simulink model "MSDR_DH_DeplV1sim"  (R2019a)
settings: Solver=ode45  StartTime=0.0  StopTime=simtime  FixedStep=0.1  MaxStep=ts_max  RelTol=rel_tolerance
values from neighbouring files (symbols this model uses):
  a_f = 1E-5*depl_fuel_temp_coef(depl_index)    [MSDR_DH_DeplV1para.m]
  a_g = 1E-5*depl_grap_temp_coef(depl_index)    [MSDR_DH_DeplV1para.m]
  A_s = 1.2245    [MSDR_DH_DeplV1para.m]
  beta = depl_beta(depl_index,:)    [MSDR_DH_DeplV1para.m]
  beta_t = sum(beta)    [MSDR_DH_DeplV1para.m]
  Cp_f = depl_Cp_Fuel_coef*1.355616e-3    [MSDR_DH_DeplV1para.m]
  Cp_p = Cp_s_shx    [MSDR_DH_DeplV1para.m]
  Cp_s = Cp_s*1e-6    (= 3.588208e-09)    [MSDR_DH_DeplV1para.m]
  Cp_sc = 4761.392e-6    (= 0.004761392)    [MSDR_DH_DeplV1para.m]
  Cp_w = 456.056e-6    (= 0.000456056)    [MSDR_DH_DeplV1para.m]
  D_it = 0.0141478    [MSDR_DH_DeplV1para.m]
  D_ot = 0.015875    [MSDR_DH_DeplV1para.m]
  DHRS_TIME_K = 10    [MSDR_DH_DeplV1para.m]
  dHs_dPs = -0.042433622114357    (= -0.0424336221144)    [MSDR_DH_DeplV1para.m]
  Epsilon = 1E-3    (= 0.001)    [MSDR_DH_DeplV1para.m]
  Fiss_factor = 2.464783802008740e-03    (= 0.00246478380201)    [MSDR_DH_DeplV1para.m]
  gamma0 = 9.635981959409105e-01    (= 0.963598195941)    [MSDR_DH_DeplV1para.m]
  gamma1 = 3.560674858154914e-02    (= 0.0356067485815)    [MSDR_DH_DeplV1para.m]
  gamma2 = 7.950554775404400e-04    (= 0.00079505547754)    [MSDR_DH_DeplV1para.m]
  gamma_I = 5.1135e-2    (= 0.051135)    [MSDR_DH_DeplV1para.m]
  gamma_Pm = 1.08E-2    (= 0.0108)    [MSDR_DH_DeplV1para.m]
  gamma_Xe = 1.1628e-2    (= 0.011628)    [MSDR_DH_DeplV1para.m]
  h_pw = h_s_shx    [MSDR_DH_DeplV1para.m]
  h_wb = 13349.334646671E-6    (= 0.0133493346467)    [MSDR_DH_DeplV1para.m]
  h_ws = 5732.378387768E-6    (= 0.00573237838777)    [MSDR_DH_DeplV1para.m]
  h_wsc = 8385.005556375E-6    (= 0.00838500555638)    [MSDR_DH_DeplV1para.m]
  hA_fg = [h_fg*A_fg/2, h_fg*A_fg/2]    [MSDR_DH_DeplV1para.m]
  hA_p_phx1 = h_p_phx*A_p_phx    [MSDR_DH_DeplV1para.m]
  hA_p_phx2 = h_p_phx*A_p_phx    [MSDR_DH_DeplV1para.m]
  hA_p_phx3 = h_p_phx*A_p_phx    [MSDR_DH_DeplV1para.m]
  hA_p_phx4 = h_p_phx*A_p_phx    [MSDR_DH_DeplV1para.m]
  hA_p_phx5 = h_p_phx*A_p_phx    [MSDR_DH_DeplV1para.m]
  hA_p_phx6 = h_p_phx*A_p_phx    [MSDR_DH_DeplV1para.m]
  hA_p_shx1 = h_p_shx*A_p_shx    [MSDR_DH_DeplV1para.m]
  hA_p_shx2 = h_p_shx*A_p_shx    [MSDR_DH_DeplV1para.m]
  hA_p_shx3 = h_p_shx*A_p_shx    [MSDR_DH_DeplV1para.m]
  hA_p_shx4 = h_p_shx*A_p_shx    [MSDR_DH_DeplV1para.m]
  hA_p_shx5 = h_p_shx*A_p_shx    [MSDR_DH_DeplV1para.m]
  hA_p_shx6 = h_p_shx*A_p_shx    [MSDR_DH_DeplV1para.m]
  hA_s_phx1 = h_s_phx*A_s_phx    [MSDR_DH_DeplV1para.m]
  hA_s_phx2 = h_s_phx*A_s_phx    [MSDR_DH_DeplV1para.m]
  hA_s_phx3 = h_s_phx*A_s_phx    [MSDR_DH_DeplV1para.m]
  hA_s_phx4 = h_s_phx*A_s_phx    [MSDR_DH_DeplV1para.m]
  hA_s_phx5 = h_s_phx*A_s_phx    [MSDR_DH_DeplV1para.m]
  hA_s_phx6 = h_s_phx*A_s_phx    [MSDR_DH_DeplV1para.m]
  hA_s_shx1 = h_s_shx*A_s_shx    [MSDR_DH_DeplV1para.m]
  hA_s_shx2 = h_s_shx*A_s_shx    [MSDR_DH_DeplV1para.m]
  hA_s_shx3 = h_s_shx*A_s_shx    [MSDR_DH_DeplV1para.m]
  hA_s_shx4 = h_s_shx*A_s_shx    [MSDR_DH_DeplV1para.m]
  hA_s_shx5 = h_s_shx*A_s_shx    [MSDR_DH_DeplV1para.m]
  hA_s_shx6 = h_s_shx*A_s_shx    [MSDR_DH_DeplV1para.m]
  I_0 = gamma_I*Sig_f_msdr*phi_0/lam_I    [MSDR_DH_DeplV1para.m]
  Ifa = [0.25, 0.25]    [MSDR_DH_DeplV1para.m]
  Ifb = [0.25, 0.25]    [MSDR_DH_DeplV1para.m]
  Ig = [0.5, 0.5]    [MSDR_DH_DeplV1para.m]
  K_1 = 11.632248097704855    (= 11.6322480977)    [MSDR_DH_DeplV1para.m]
  K_4 = b(1)    [MSDR_DH_DeplV1para.m]
  K_5 = a(1)    [MSDR_DH_DeplV1para.m]
  K_b = 12.834854076292217    (= 12.8348540763)    [MSDR_DH_DeplV1para.m]
  K_pump = 1/5    (= 0.2)    [MSDR_DH_DeplV1para.m]
  K_sc = -17.615718797133468    (= -17.6157187971)    [MSDR_DH_DeplV1para.m]
  ka = [0.235, 0.235]    [MSDR_DH_DeplV1para.m]
  kb = [0.235, 0.235]    [MSDR_DH_DeplV1para.m]
  kga = [0.015, 0.015]    [MSDR_DH_DeplV1para.m]
  kgb = [0.015, 0.015]    [MSDR_DH_DeplV1para.m]
  L = 8.5344    [MSDR_DH_DeplV1para.m]
  L_b = 2.3645    [MSDR_DH_DeplV1para.m]
  L_s = 4.723    [MSDR_DH_DeplV1para.m]
  Lam = depl_Lam(depl_index)    [MSDR_DH_DeplV1para.m]
  lam = [1.240E-02, 3.05E-02, 1.11E-01, 3.01E-01, 1.140E+00, 3.014E+00]    [MSDR_DH_DeplV1para.m]
  lam_bubl = 2.0e-2    (= 0.02)    [MSDR_DH_DeplV1para.m]
  lam_I = 2.875e-5    (= 2.875e-05)    [MSDR_DH_DeplV1para.m]
  lam_Pm = log(2)/(2.21*24*3600)    [MSDR_DH_DeplV1para.m]
  lam_Xe = 2.0916e-5    (= 2.0916e-05)    [MSDR_DH_DeplV1para.m]
  lambda0 = 0.0945298    [MSDR_DH_DeplV1para.m]
  lambda1 = 0.00441957    [MSDR_DH_DeplV1para.m]
  lambda2 = 8.60979e-05    [MSDR_DH_DeplV1para.m]
  m_3m = W_3*2    (= 8618.207327)    [MSDR_DH_DeplV1para.m]
  m_f_t = total_mp_phx + core_fm + mp_phxm*3 + m_fm    [MSDR_DH_DeplV1para.m]
  m_fm = W_f*1    (= 4989.48)    [MSDR_DH_DeplV1para.m]
  M_stm = 0.018    [MSDR_DH_DeplV1para.m]
  mcp_fa = mfa*Cp_f    [MSDR_DH_DeplV1para.m]
  mcp_fb = mfb*Cp_f    [MSDR_DH_DeplV1para.m]
  mcp_g = mg*Cp_g    [MSDR_DH_DeplV1para.m]
  mcp_p_phx1 = Cp_p_phx*mp_phx1    [MSDR_DH_DeplV1para.m]
  mcp_p_phx2 = Cp_p_phx*mp_phx2    [MSDR_DH_DeplV1para.m]
  mcp_p_phx3 = Cp_p_phx*mp_phx3    [MSDR_DH_DeplV1para.m]
  mcp_p_phx4 = Cp_p_phx*mp_phx4    [MSDR_DH_DeplV1para.m]
  mcp_p_phx5 = Cp_p_phx*mp_phx5    [MSDR_DH_DeplV1para.m]
  mcp_p_phx6 = Cp_p_phx*mp_phx6    [MSDR_DH_DeplV1para.m]
  mcp_p_shx1 = Cp_p_shx*mp_shx1    [MSDR_DH_DeplV1para.m]
  mcp_p_shx2 = Cp_p_shx*mp_shx2    [MSDR_DH_DeplV1para.m]
  mcp_p_shx3 = Cp_p_shx*mp_shx3    [MSDR_DH_DeplV1para.m]
  mcp_p_shx4 = Cp_p_shx*mp_shx4    [MSDR_DH_DeplV1para.m]
  mcp_p_shx5 = Cp_p_shx*mp_shx5    [MSDR_DH_DeplV1para.m]
  mcp_p_shx6 = Cp_p_shx*mp_shx6    [MSDR_DH_DeplV1para.m]
  mcp_s_phx1 = Cp_s_phx*ms_phx1    [MSDR_DH_DeplV1para.m]
  mcp_s_phx2 = Cp_s_phx*ms_phx2    [MSDR_DH_DeplV1para.m]
  mcp_s_phx3 = Cp_s_phx*ms_phx3    [MSDR_DH_DeplV1para.m]
  mcp_s_phx4 = Cp_s_phx*ms_phx4    [MSDR_DH_DeplV1para.m]
  mcp_s_phx5 = Cp_s_phx*ms_phx5    [MSDR_DH_DeplV1para.m]
  mcp_s_phx6 = Cp_s_phx*ms_phx6    [MSDR_DH_DeplV1para.m]
  mcp_s_shx1 = Cp_s_shx*ms_shx1    [MSDR_DH_DeplV1para.m]
  mcp_s_shx2 = Cp_s_shx*ms_shx1    [MSDR_DH_DeplV1para.m]
  mcp_s_shx3 = Cp_s_shx*ms_shx1    [MSDR_DH_DeplV1para.m]
  mcp_s_shx4 = Cp_s_shx*ms_shx1    [MSDR_DH_DeplV1para.m]
  mcp_s_shx5 = Cp_s_shx*ms_shx1    [MSDR_DH_DeplV1para.m]
  mcp_s_shx6 = Cp_s_shx*ms_shx1    [MSDR_DH_DeplV1para.m]
  mcp_t_phx1 = Cp_t_phx*mt_phx1    [MSDR_DH_DeplV1para.m]
  mcp_t_phx2 = Cp_t_phx*mt_phx2    [MSDR_DH_DeplV1para.m]
  mcp_t_phx3 = Cp_t_phx*mt_phx3    [MSDR_DH_DeplV1para.m]
  mcp_t_phx4 = Cp_t_phx*mt_phx4    [MSDR_DH_DeplV1para.m]
  mcp_t_phx5 = Cp_t_phx*mt_phx5    [MSDR_DH_DeplV1para.m]
  mcp_t_phx6 = Cp_t_phx*mt_phx6    [MSDR_DH_DeplV1para.m]
  mcp_t_shx1 = Cp_t_phx*mt_shx1    [MSDR_DH_DeplV1para.m]
  mcp_t_shx2 = Cp_t_phx*mt_shx2    [MSDR_DH_DeplV1para.m]
  mcp_t_shx3 = Cp_t_phx*mt_shx3    [MSDR_DH_DeplV1para.m]
  mcp_t_shx4 = Cp_t_phx*mt_shx4    [MSDR_DH_DeplV1para.m]
  mcp_t_shx5 = Cp_t_phx*mt_shx5    [MSDR_DH_DeplV1para.m]
  mcp_t_shx6 = Cp_t_phx*mt_shx6    [MSDR_DH_DeplV1para.m]
  ... (+159 more)
undefined symbols (not defined in the file or in its folder): C0, DHRS_MODE, DHRS_Power, DHRS_time, ln, P, Trip_P1_pump, Trip_P2_pump, Trip_P3_pump, Trip_S1_pump, Trip_S2_pump, Trip_S3_pump, Trip_T1_pump, Trip_T2_pump, Trip_T3_pump, Trip_UHX
libraries: simulink x2
(part 4 of 4)

== system MSDR_DH_DeplV1sim/SECONDARY SIDE/Variant Subsystem/UHX/UHX ==
  HITEC_INLET : Inport
  HITEC_FLOW_FRAC : Inport  Port=2
  Enable : EnablePort
  Demand From Workspace : FromWorkspace  VariableName=demand  SampleTime=1  Interpolate=off  OutputAfterFinalValue=Holding final value
  Mux2 : Mux  Inputs=9
      settings: DisplayOption=signals
  Tp1_otsg : Integrator  InitialCondition=100
  Tp2_otsg : Integrator  InitialCondition=T_p2
  Tp3_otsg : Integrator  InitialCondition=T_p3
  Tp4_otsg : Integrator  InitialCondition=T_p4
  Tp5_otsg : Integrator  InitialCondition=T_p5
  Tp6_otsg : Integrator  InitialCondition=T_p6
  d(Tp1_UHX)/dt : Fcn  Expr=(u[2]*W_3/mn_UHX)*(u[1]-u[4]) - (u[3]*P/n_UHX)/(mn_UHX*Cp_p)
  d(Tp2_UHX)/dt : Fcn  Expr=(u[2]*W_3/mn_UHX)*(u[4]-u[5]) - (u[3]*P/n_UHX)/(mn_UHX*Cp_p)
  d(Tp3_UHX)/dt : Fcn  Expr=(u[2]*W_3/mn_UHX)*(u[5]-u[6]) - (u[3]*P/n_UHX)/(mn_UHX*Cp_p)
  d(Tp4_UHX)/dt : Fcn  Expr=(u[2]*W_3/mn_UHX)*(u[6]-u[7]) - (u[3]*P/n_UHX)/(mn_UHX*Cp_p)
  d(Tp5_UHX)/dt : Fcn  Expr=(u[2]*W_3/mn_UHX)*(u[7]-u[8]) - (u[3]*P/n_UHX)/(mn_UHX*Cp_p)
  d(Tp6_UHX)/dt : Fcn  Expr=(u[2]*W_3/mn_UHX)*(u[8]-u[9]) - (u[3]*P/n_UHX)/(mn_UHX*Cp_p)
  HITEC_OUTLET : Outport
  wires:
  Tp2_otsg/1 -> Mux2/5
  HITEC_INLET/1 -> Mux2/1
  Mux2/1 -> d(Tp1_UHX)/dt/1, d(Tp2_UHX)/dt/1, d(Tp3_UHX)/dt/1, d(Tp4_UHX)/dt/1, d(Tp5_UHX)/dt/1, d(Tp6_UHX)/dt/1
  d(Tp4_UHX)/dt/1 -> Tp4_otsg/1
  d(Tp1_UHX)/dt/1 -> Tp1_otsg/1
  Tp4_otsg/1 -> Mux2/7
  d(Tp2_UHX)/dt/1 -> Tp2_otsg/1
  d(Tp3_UHX)/dt/1 -> Tp3_otsg/1
  Tp5_otsg/1 -> Mux2/8
  d(Tp5_UHX)/dt/1 -> Tp5_otsg/1
  Demand From Workspace/1 -> Mux2/3
  Tp6_otsg/1 -> HITEC_OUTLET/1, Mux2/9
  HITEC_FLOW_FRAC/1 -> Mux2/2
  d(Tp6_UHX)/dt/1 -> Tp6_otsg/1
  Tp1_otsg/1 -> Mux2/4
  Tp3_otsg/1 -> Mux2/6
